simulink model "RuleBasedAlgo_sfunc"  (R2018b)
settings: Solver=ode2  StartTime=0.0  StopTime=inf  FixedStep=t_step  RelTol=1e-3
libraries: pil_lib x1
settings Model: Creator=Aman-Home  LastModifiedBy=Aman-Home

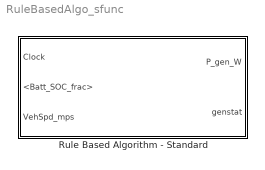
== system RuleBasedAlgo_sfunc ==
  Rule Based Algorithm - Standard : Subsystem  DialogController=pil_create_dialog  LoadFcn=|
      | try
      |    if ~strcmp(rtw.pil.getPILVersion, '9.5 (R2018b)_13')
      |       set_param(gcb, 'DialogController', '');
      |       set_param(gcb, 'DialogControllerArgs', '');
      |    end
      | catch e
      |       set_param(gcb, 'DialogController', '');
      |       set_param(gcb, 'DialogControllerArgs', '');
      | end
      mask help: PIL:pil:XILBlockMaskDesc
      mask Display: disp('SIL');

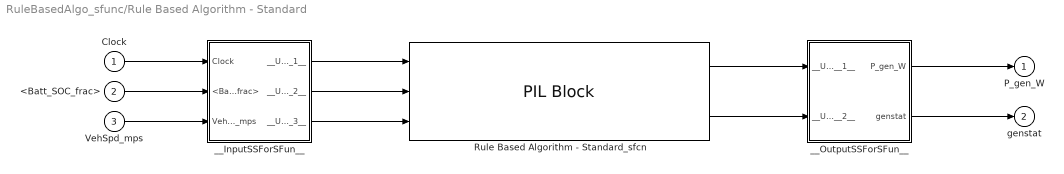
== system RuleBasedAlgo_sfunc/Rule Based Algorithm - Standard ==
  Clock : Inport
  <Batt_SOC_frac> : Inport  Port=2
  VehSpd_mps : Inport  Port=3
  Rule Based Algorithm - Standard_sfcn : pil_lib/PIL Block  SimulationMode=SIL  IsTopModelPIL=off  CodeDir=C:\Users\Aman-Home\Documents\MATLAB\DocResWork\Simulation_Models\SHEV_Model\Rule_ert_rtw  AnchorDir=C:\Users\Aman-Home\Documents\MATLAB\DocResWork\Simulation_Models\SHEV_Model  ConfigName=Software-in-the-Loop (SIL)  XrelIsTopModelCode=on  XrelIsReusable=off  XrelDWorkNames={}  XrelDWorkTypes={}  XrelModelArgVals={}  XrelOrderedParamNames={}
  __InputSSForSFun__ : Subsystem
  __OutputSSForSFun__ : Subsystem
  P_gen_W : Outport
  genstat : Outport  Port=2
  wires:
  Clock/1 -> __InputSSForSFun__/1(Clock)
  <Batt_SOC_frac>/1 -> __InputSSForSFun__/2(<Batt_SOC_frac>)
  VehSpd_mps/1 -> __InputSSForSFun__/3(VehSpd_mps)
  __InputSSForSFun__/1(__UniqueOutportName__1__) -> Rule Based Algorithm - Standard_sfcn/1
  __InputSSForSFun__/2(__UniqueOutportName__2__) -> Rule Based Algorithm - Standard_sfcn/2
  __InputSSForSFun__/3(__UniqueOutportName__3__) -> Rule Based Algorithm - Standard_sfcn/3
  Rule Based Algorithm - Standard_sfcn/1 -> __OutputSSForSFun__/1(__UniqueInportName__1__)
  Rule Based Algorithm - Standard_sfcn/2 -> __OutputSSForSFun__/2(__UniqueInportName__2__)
  __OutputSSForSFun__/1(P_gen_W) -> P_gen_W/1
  __OutputSSForSFun__/2(genstat) -> genstat/1

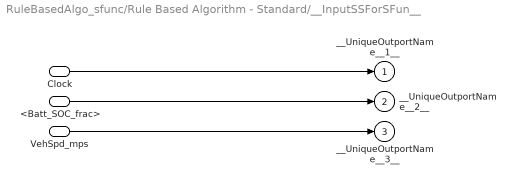
== system RuleBasedAlgo_sfunc/Rule Based Algorithm - Standard/__InputSSForSFun__ ==
  Clock : Inport
  <Batt_SOC_frac> : Inport  Port=2
  VehSpd_mps : Inport  Port=3
  __UniqueOutportName__1__ : Outport
  __UniqueOutportName__2__ : Outport  Port=2
  __UniqueOutportName__3__ : Outport  Port=3
  wires:
  Clock/1 -> __UniqueOutportName__1__/1
  <Batt_SOC_frac>/1 -> __UniqueOutportName__2__/1
  VehSpd_mps/1 -> __UniqueOutportName__3__/1

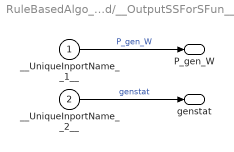
== system RuleBasedAlgo_sfunc/Rule Based Algorithm - Standard/__OutputSSForSFun__ ==
  __UniqueInportName__1__ : Inport
  __UniqueInportName__2__ : Inport  Port=2
  P_gen_W : Outport
  genstat : Outport  Port=2
  wires:
  __UniqueInportName__1__/1 -> P_gen_W/1  "P_gen_W"
  __UniqueInportName__2__/1 -> genstat/1  "genstat"
